simulink model "HydrogenRefuelingStation_Param"  (R2023b)
settings: Solver=VariableStepAuto  StartTime=0.0  StopTime=finSimulation  RelTol=1e-3  AbsTol=1e-3
PreLoadFcn:
  | load hydrogen_properties.mat
  | load silicone_fluid_properties.mat
  | 
  | p_storage = 200; % [bar]
  | p_vehicle_init = 100; % [bar]
  | T_env = 25; % [degC]
  | T_fluid = -60; % [degC]
  | 
  | V_vehicle = 172; % [l]
  | 
  | tube_D = 0.04; % [m]
  | hose_D = 0.0064; % [m]
  | pipe_D = 0.1; % [m]
  | 
  | num_buffer = 2;
  | 
  | intercooler_num_tubes = 25;
  | intercooler_tube_D = 0.008; % [m]
  | intercooler_shell_D = 0.1; % [m]
  | intercooler_L = 2; % [m]
  | 
  | precooler_tube_W = 0.001; % [m]
  | precooler_num_tubes = 50*25;
  | precooler_L = 1; % [m]
values from neighbouring files (symbols this model uses):
  EngDemandTime = 3000    [launch.m]
  EngThrottle = 1    [launch.m]
  ext_bufferEng_D = 0.025    [System_Parameters.m]
  ext_Manifold_D = 0.007    [System_Parameters.m]
  ext_vehTank_D = 0.25    [System_Parameters.m]
  in_bufferEng_D = 0.0064    [System_Parameters.m]
  in_Eng_D = 0.0064    [System_Parameters.m]
  in_Man_D = 0.0064    [System_Parameters.m]
  inOut_vehTank_D = 0.0064    [System_Parameters.m]
  int_bufferEng_D = 0.024    [System_Parameters.m]
  int_Manifold_D = 0.0064    [System_Parameters.m]
  int_vehTank_D = 0.22    [System_Parameters.m]
  L_bufferEng = 1    [System_Parameters.m]
  L_Manifold = 1    [System_Parameters.m]
  L_vehTank = 2    [System_Parameters.m]
  MV_D = 0.0064    [System_Parameters.m]
  out_bufferEng_D = 0.0064/2    (= 0.0032)    [System_Parameters.m]
  out_Eng_D = 0.0064    [System_Parameters.m]
  out_Man_D = 0.0064    [System_Parameters.m]
  Pipe_ConnMan_D = 0.0064    [System_Parameters.m]
  Pipe_ManPR_D = 0.0064    [System_Parameters.m]
  Pipe_ManTank_D = 0.0064    [System_Parameters.m]
  Pipe_PRBuffer_D = 0.0064    [System_Parameters.m]
  redn_PR_D = 0.0064    [System_Parameters.m]
  redn_PR_setP = 160    [System_Parameters.m]
  relief_PR_D = 0.0064    [System_Parameters.m]
  relief_vehTank_D = 0.0064    [System_Parameters.m]
  silicone_fluid =     [silicone_fluid_properties.mat]
  statConn_D = 0.0064    [System_Parameters.m]
  stationTrigger_Time = 2400    [System_Parameters.m]
  SV_D = 0.0064    [System_Parameters.m]
  tank_Man_D = 0.0064    [System_Parameters.m]
  TempCont_vehTank_D = 0.0064    [System_Parameters.m]
  vehConn_D = 0.0064    [System_Parameters.m]
  WP_high = 700    [System_Parameters.m]
libraries: fl_lib x128, nesl_utility x60, SimscapeFluids_lib x41, slpidlib x4
(part 1 of 6)
CloseFcn:
  | try,close(h1_HydrogenRefuelingStation),end
  | clear h1_HydrogenRefuelingStation
  | try,close(h2_HydrogenRefuelingStation),end
  | clear h2_HydrogenRefuelingStation
  | try,close(h3_HydrogenRefuelingStation),end
  | clear h3_HydrogenRefuelingStation
  | 
  | clear tout simlog_HydrogenRefuelingStation
  | clear H2 silicone_fluid
  | clear p_storage p_vehicle_init T_env T_fluid
  | clear V_vehicle tube_D hose_D pipe_D num_buffer
  | clear intercooler_num_tubes intercooler_tube_D intercooler_shell_D intercooler_L
  | clear precooler_tube_W precooler_num_tubes precooler_L
Description:
  | Hydrogen Refueling Station
settings Model: Creator=The MathWorks, Inc.  LastModifiedBy=sb74808
settings SolverCC: AutoScaleAbsTol=off  ZeroCrossAlgorithm=Adaptive  AlgebraicLoopSolver=TrustRegion  MaxZcPerStep=1
settings DataIOCC: ReturnWorkspaceOutputs=off
settings DebuggingCC: IgnoredZcDiagnostic=none  UnconnectedInputMsg=warning  UnconnectedOutputMsg=warning  UnconnectedLineMsg=warning  SymbolicDimsDataTypeCodeGenerationDiagnostic=none
settings ModelReferenceCC: EnableRefExpFcnMdlSchedulingChecks=on
settings SFSimCC: CustomCodeUndefinedFunction=UseInterfaceOnly
settings RTWCC: DLArmComputeVersion=19.05
settings SimscapeCC: SimscapeLogType=all  SimscapeLogSimulationStatistics=on  SimscapeLogName=simlog_HydrogenRefuelingStation  SimscapeLogDataHistory=10000

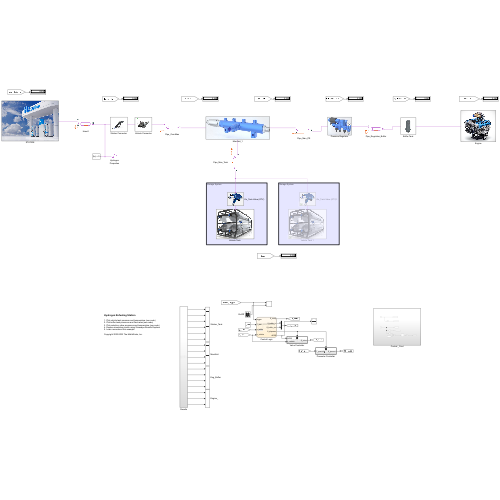
[thumbnail: Simulink's stored preview of the top-level diagram]
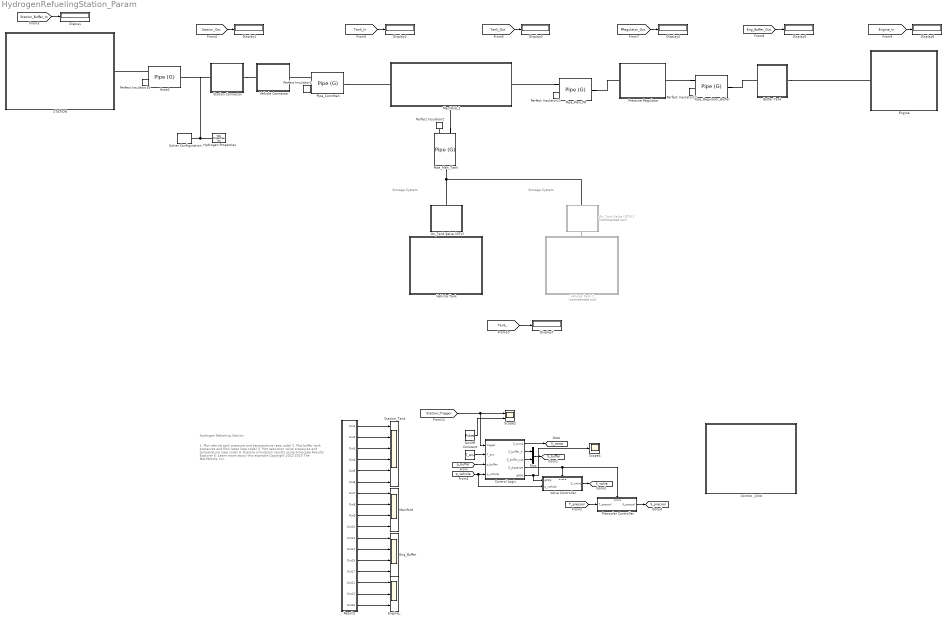
== system HydrogenRefuelingStation_Param ==
  note: Storage System
  note: Hydrogen Refueling Station
  note: 1. Plot vehicle tank pressure and temperature (see code)
      | 2. Plot buffer tank pressures and flow rates (see code)
      | 3. Plot reduction valve pressures and temperature (see code)
      | 4. Explore simulation results using Simscape Results Explorer
      | 5. Learn more about this example
      |
      | Copyright 2022-2023 The MathWorks, Inc.
  note: Storage System
  Buffer Tank : Subsystem
      mask Display: image('BufferTanks.png');
  Constant : Constant  Value=T_env
  Control Logic : Stateflow chart  Tag=PublishSubsystem  TreatAsAtomicUnit=on
      settings: PortSchema="{\"entries\":[{\"content\":{\"sides\":[{\"content\":{\"connectorIds\":[\"In4\",\"In1\",\"In2\",\"In3\"]},\"type\":\"ConnectorPlacement.EquallySpacedRectSide\",\"uuid\":\"229b392f-68ea-49e2-87d9-89899b0a8cf1\"},{\"content\":{\"connectorIds\":[\"Out2\",\"Out4\",\"Out5\",\"Out3\",\"Out1\"],\"side\":\"RIGHT\"},\"type\":\"ConnectorPlacement.EquallySpacedRectSide\",\"uuid\":\"67ffe3ee-1dc5-488d-9b3d-4fb771a503f6\"},{\"content\":{\"connectorIds\":[],\"side\":\"TOP\"},\"type\":\"ConnectorPlacement.EquallySpacedRectSide\",\"uuid\":\"803859aa-a920-419c-845f-f763b20f74de\"}]},\"type\":\"ConnectorPlacement.EquallySpacedConnector\",\"uuid\":\"a5c406d3-0f1f-4c42-8168-eaeee8551f27\"}],\"packageUris\":[\"http://schema.mathworks.com/mf0/Connector/R2020b\"],\"version\":\"1.0\"}"
  Control _Cmd : Subsystem
  Display{,1..7} (8 alike) : Display
  Eng_Buffer : Scope  NumInputPorts=4
  Engine : Subsystem
      mask Display: image('Engine_H2.PNG');
  Engine_ : Scope  NumInputPorts=3
  Hose2 : fl_lib/Gas/Elements/Pipe (G)  length=4 m  area=pi*statConn_D^2/4 m^2  Dh=statConn_D m  length_add=0.6 m  roughness=15e-6 m  Re_lam=2000  Re_tur=4000  shape_factor=64  Nu_lam=3.66  p_I_specify=on  p_I_priority=High  p_I=p_vehTank_init bar  p_I_nominal_specify=off  p_I_nominal_unit=MPa  p_I_nominal_value=1  T_I_specify=on  T_I_priority=High  T_I=T_env degC  T_I_nominal_specify=off  T_I_nominal_unit=K  T_I_nominal_value=1  rho_I_specify=off  rho_I_priority=None  rho_I=1.2 kg/m^3  rho_I_nominal_specify=off  rho_I_nominal_unit=kg/m^3  rho_I_nominal_value=1
  Hydrogen Properties : fl_lib/Gas/Utilities/Gas Properties (G)  gas_spec=foundation.enum.gas_spec.real_gas  R=0.287 kJ/(K*kg)  Z=1  T_ref=293.15 K  h_ref=420 kJ/kg  cp_ref=1 kJ/(K*kg)  mu_ref=18 s*uPa  k_ref=26 mW/(K*m)  T_TLU1=[150 : 10 : 200, 250 : 50 : 1000, 1500, 2000]' K  h_TLU1=[275.264783730547; 285.377054177734; 295.474578903607; 305.560871069627; 315.638490783961; 325.709373787179; 376.008033649461; 426.297784741196; 476.678788323875; 527.253890684429; 578.12722735187; 629.395040865183; 681.137690131207; 733.415442873049; 786.267894376777; 839.715851152006; 893.764459999509; 948.406676876931; 1003.62653219711; 1059.40193232821; 1115.70691941005; 1172.51341226958; 1762.18512007361; 2377.14064127409] kJ/kg  cp_TLU1=[1.01211492398124; 1.01042105529234; 1.00914159006373; 1.00815898273273; 1.00739688341918; 1.00680484569075; 1.00554191216852; 1.00637389921747; 1.0092105862442; 1.01414404435034; 1.02111299587909; 1.02986878923959; 1.04003820504128; 1.05120320041448; 1.06296312852444; 1.07497111709439; 1.08694865668905; 1.0986858495625; 1.11003396604319; 1.12089493621399; 1.13121051694521; 1.14095251451866; 1.21001953144; 1.24628356718428] kJ/(K*kg)  mu_TLU1=[10.3766056544352; 10.9908682444892; 11.5932000841352; 12.1841060353213; 12.764067709023; 13.3335437107148; 16.038149065057; 18.5373404836509; 20.8671495114253; 23.0554226800681; 25.1239717991959; 27.0901379793485; 28.96790749834; 30.7687111230031; 32.5020036481173; 34.17569027566; 35.7964450415303; 37.3699520751368; 38.9010908824946; 40.3940804368247; 41.8525925389218; 43.279841956487; 56.3254722619962; 68.068290080945] s*uPa  k_TLU1=[14.1517155766309; 15.0474512994325; 15.9300520513026; 16.7998749295306; 17.6573089963228; 18.5027588910197; 22.5644026699512; 26.384465676638; 30.0032801168886; 33.4532006033488; 36.7600619429332; 39.9446251241844; 43.0237448740114; 46.0112537033799; 48.9186234516389; 51.7554617696538; 54.5298878921773; 57.2488200454925; 59.9181976996146; 62.5431553064749; 65.128159527924; 67.6771186900213; 91.7815514375552; 114.486299090693] mW/(K*m)  T_TLU2=H2.T K  p_TLU2=H2.p MPa  rho_TLU2=H2.rho kg/m^3  s_TLU2=H2.s kJ/(K*kg)  h_TLU2=H2.h kJ/kg  cp_TLU2=H2.cp kJ/(K*kg)  mu_TLU2=H2.mu s*uPa  k_TLU2=H2.k mW/(K*m)  beta_TLU2=H2.beta MPa  alpha_TLU2=H2.alpha 1/K  T_min_perfect=1 K  T_max_perfect=inf K  p_min_perfect=1 Pa  p_max_perfect=inf MPa  T_range_flag=foundation.enum.T_range_G.from_props  T_min_semiperfect=150 K  T_max_semiperfect=2000 K  p_min_semiperfect=1 Pa  p_max_semiperfect=inf MPa  pT_region_flag=foundation.enum.pT_region_G.from_props  pT_validity_TLU2=ones(24, 20)  T_min_real=150 K  T_max_real=2000 K  p_min_real=0.001 MPa  p_max_real=10 MPa  p_atm=0.101325 MPa  properties_range_check=simscape.enum.assert.action.error  Mach_rev=0.001 / 10
  Manifold : Scope  NumInputPorts=4
  Manifold_1 : Subsystem  Tag=PublishSubsystem
      settings: PortSchema="{\"entries\":[{\"content\":{\"sides\":[{\"content\":{\"connectorIds\":[\"LConn1\"]},\"type\":\"ConnectorPlacement.EquallySpacedRectSide\",\"uuid\":\"b00ba4dd-6dda-4fc1-8418-16d977b72658\"},{\"content\":{\"connectorIds\":[\"RConn1\"],\"side\":\"RIGHT\"},\"type\":\"ConnectorPlacement.EquallySpacedRectSide\",\"uuid\":\"8ce3b878-20da-4ae3-b32b-b25a417e40c7\"},{\"content\":{\"side\":\"TOP\"},\"type\":\"ConnectorPlacement.EquallySpacedRectSide\",\"uuid\":\"178fea87-568c-460e-ad58-627cda0af208\"},{\"content\":{\"connectorIds\":[\"RConn2\"],\"side\":\"BOTTOM\"},\"type\":\"ConnectorPlacement.EquallySpacedRectSide\",\"uuid\":\"da377dea-32af-4e40-bf21-9605c244d1e1\"}]},\"type\":\"ConnectorPlacement.EquallySpacedConnector\",\"uuid\":\"9a70e3bb-46a6-4db7-b9e8-afd83bfe5c73\"}],\"packageUris\":[\"http://schema.mathworks.com/mf0/Connector/R2020b\"],\"version\":\"1.0\"}"
      mask Display: image('Manifold.jpg');
  Mux : Mux  Inputs=2
  On/Off : DiscretePulseGenerator  PulseType=Time based  Period=3600  PulseWidth=300 / 3600 * 100  PhaseDelay=2400
  On_Tank Valve (OTV) : Subsystem
      settings: PortSchema="{\"entries\":[{\"content\":{\"sides\":[{\"content\":{},\"type\":\"ConnectorPlacement.EquallySpacedRectSide\",\"uuid\":\"9d4661ff-bfd9-4877-b119-c7ad3b9158b6\"},{\"content\":{\"side\":\"RIGHT\"},\"type\":\"ConnectorPlacement.EquallySpacedRectSide\",\"uuid\":\"403ca504-bf4e-462a-96fb-b4ae1a4b51b2\"},{\"content\":{\"connectorIds\":[\"LConn1\"],\"side\":\"TOP\"},\"type\":\"ConnectorPlacement.EquallySpacedRectSide\",\"uuid\":\"f4930e4d-a2e3-4901-b32b-f7ec2035bb63\"},{\"content\":{\"connectorIds\":[\"RConn1\"],\"side\":\"BOTTOM\"},\"type\":\"ConnectorPlacement.EquallySpacedRectSide\",\"uuid\":\"d9d264b6-0917-42e9-93e5-2bb8167430bf\"}]},\"type\":\"ConnectorPlacement.EquallySpacedConnector\",\"uuid\":\"c2399e2b-f5dd-4ca5-8bb9-d4f6c8dace36\"}],\"packageUris\":[\"http://schema.mathworks.com/mf0/Connector/R2020b\"],\"version\":\"1.0\"}"
      mask Display: image('OTV.png');
  On_Tank Valve (OTV)1 : Subsystem  Commented=on
      settings: PortSchema="{\"entries\":[{\"content\":{\"sides\":[{\"content\":{},\"type\":\"ConnectorPlacement.EquallySpacedRectSide\",\"uuid\":\"9d4661ff-bfd9-4877-b119-c7ad3b9158b6\"},{\"content\":{\"side\":\"RIGHT\"},\"type\":\"ConnectorPlacement.EquallySpacedRectSide\",\"uuid\":\"403ca504-bf4e-462a-96fb-b4ae1a4b51b2\"},{\"content\":{\"connectorIds\":[\"LConn1\"],\"side\":\"TOP\"},\"type\":\"ConnectorPlacement.EquallySpacedRectSide\",\"uuid\":\"f4930e4d-a2e3-4901-b32b-f7ec2035bb63\"},{\"content\":{\"connectorIds\":[\"RConn1\"],\"side\":\"BOTTOM\"},\"type\":\"ConnectorPlacement.EquallySpacedRectSide\",\"uuid\":\"d9d264b6-0917-42e9-93e5-2bb8167430bf\"}]},\"type\":\"ConnectorPlacement.EquallySpacedConnector\",\"uuid\":\"c2399e2b-f5dd-4ca5-8bb9-d4f6c8dace36\"}],\"packageUris\":[\"http://schema.mathworks.com/mf0/Connector/R2020b\"],\"version\":\"1.0\"}"
      mask Display: image('OTV.png');
  Perfect Insulator{1..2,10..12} (5 alike) : fl_lib/Thermal/Thermal Elements/Perfect Insulator  T_specify=off  T_priority=None  T=293.15 K  T_nominal_specify=off  T_nominal_unit=K  T_nominal_value=1
  Pipe_ConnMan : fl_lib/Gas/Elements/Pipe (G)  length=Pipe_ConnMan_L m  area=pi*Pipe_ConnMan_D^2/4 m^2  Dh=Pipe_ConnMan_D m  length_add=0.6 m  roughness=15e-6 m  Re_lam=2000  Re_tur=4000  shape_factor=64  Nu_lam=3.66  p_I_specify=on  p_I_priority=High  p_I=p_vehTank_init bar  p_I_nominal_specify=off  p_I_nominal_unit=MPa  p_I_nominal_value=1  T_I_specify=on  T_I_priority=High  T_I=T_env degC  T_I_nominal_specify=off  T_I_nominal_unit=K  T_I_nominal_value=1  rho_I_specify=off  rho_I_priority=None  rho_I=1.2 kg/m^3  rho_I_nominal_specify=off  rho_I_nominal_unit=kg/m^3  rho_I_nominal_value=1
  Pipe_Man_PR : fl_lib/Gas/Elements/Pipe (G)  length=Pipe_ManPR_L m  area=pi*Pipe_ManPR_D^2/4 m^2  Dh=Pipe_ManPR_D m  length_add=0.6 m  roughness=15e-6 m  Re_lam=2000  Re_tur=4000  shape_factor=64  Nu_lam=3.66  p_I_specify=on  p_I_priority=High  p_I=p_vehTank_init bar  p_I_nominal_specify=off  p_I_nominal_unit=MPa  p_I_nominal_value=1  T_I_specify=on  T_I_priority=High  T_I=T_env degC  T_I_nominal_specify=off  T_I_nominal_unit=K  T_I_nominal_value=1  rho_I_specify=off  rho_I_priority=None  rho_I=1.2 kg/m^3  rho_I_nominal_specify=off  rho_I_nominal_unit=kg/m^3  rho_I_nominal_value=1
  Pipe_Man_Tank : fl_lib/Gas/Elements/Pipe (G)  length=Pipe_ManTank_L m  area=pi*Pipe_ManTank_D^2/4 m^2  Dh=Pipe_ManTank_D m  length_add=0.6 m  roughness=15e-6 m  Re_lam=2000  Re_tur=4000  shape_factor=64  Nu_lam=3.66  p_I_specify=on  p_I_priority=High  p_I=p_vehTank_init bar  p_I_nominal_specify=off  p_I_nominal_unit=MPa  p_I_nominal_value=1  T_I_specify=on  T_I_priority=High  T_I=T_env degC  T_I_nominal_specify=off  T_I_nominal_unit=K  T_I_nominal_value=1  rho_I_specify=off  rho_I_priority=None  rho_I=1.2 kg/m^3  rho_I_nominal_specify=off  rho_I_nominal_unit=kg/m^3  rho_I_nominal_value=1
  Pipe_Regulator_Buffer : fl_lib/Gas/Elements/Pipe (G)  length=Pipe_PRBuffer_L m  area=pi*Pipe_PRBuffer_D^2/4 m^2  Dh=Pipe_PRBuffer_D m  length_add=0.6 m  roughness=15e-6 m  Re_lam=2000  Re_tur=4000  shape_factor=64  Nu_lam=3.66  p_I_specify=on  p_I_priority=High  p_I=p_vehTank_init bar  p_I_nominal_specify=off  p_I_nominal_unit=MPa  p_I_nominal_value=1  T_I_specify=on  T_I_priority=High  T_I=T_env degC  T_I_nominal_specify=off  T_I_nominal_unit=K  T_I_nominal_value=1  rho_I_specify=off  rho_I_priority=None  rho_I=1.2 kg/m^3  rho_I_nominal_specify=off  rho_I_nominal_unit=kg/m^3  rho_I_nominal_value=1
  Precooler Controller : Subsystem  Tag=PublishSubsystem  TreatAsAtomicUnit=on
  Pressure Regulator : Subsystem
      mask Display: image('PressureRegulator.jpg');
  Results : Subsystem
  STATION : Subsystem
      mask Display: image('Hydrogen_Station_.png');
  Scope2 : Scope  NumInputPorts=2
  Scope4 : Scope
  Solver Configuration : nesl_utility/Solver Configuration  PhysicalDomain=network_engine_domain  SubClassName=solver  LeftPortType=input  RightPortType=generic  Tones=[]  Harmonics=[]  SimulateNoise=off  Profile=off  UseLocalSampling=off  EnableSwitchedLinearOptims=on  FrequencyDomain=off  UseCCode=off  RelTol=0.001  AbsTol=0.001  MinStep=1e-09  ToWorkspace=off  RevertToSquareIcSolve=off  NumHomotopyIterations=100  PhasorMode=off  PhasorModeNumHarmonics=1  ConsistencySolver=NEWTON_XTOL_AFTER_FTOL  IndexReductionMethod=DerivativeReplacement  DoDC=off  ResidualTolerance=1e-09  ConsistencyTolSource=GLOBAL  ConsistencyAbsTol=0.001  ConsistencyRelTol=0.001  ConsistencyTolFactor=0.001  UseLocalSolver=off  LocalSolverChoice=NE_BACKWARD_EULER_ADVANCER  ResolveIndetEquations=on  FunctionEvalNumThread=1  LocalSolverSampleTime=0.001  DoFixedCost=off  MaxNonlinIter=3  MaxModeIter=2  ComputeImpulses=off  ImpulseIterations=2  LinearAlgebra=auto  LinearAlgebraNumThread=0  EquationFormulation=NE_TIME_EF  DelaysMemoryBudget=1024  AutomaticFiltering=on  FilteringTimeConstant=0.001  PartitionStorageMethod=AS_NEEDED  PartitionMemoryBudget=1024  PartitionMethod=ROBUST  MultibodyUseLocalSolver=off  MultibodyLocalSolverChoice=ODE1  MultibodyLocalSolverSampleTime=0.001
  Station Connector : Subsystem
      mask Display: image('FuelingNozzle.png');
  Station_Tank : Scope  NumInputPorts=6
  Valve Controller : Subsystem  Tag=PublishSubsystem  TreatAsAtomicUnit=on
  Vehicle Connector : Subsystem
      mask Display: image('Veh_Connector.jpg');
  "Vehicle Tank " : Subsystem
      mask Display: image('Vehicle_Tank.png');
  Vehicle Tank 1 : Subsystem  Commented=on
      mask Display: image('Vehicle_Tank.png');
  tag scope: S_buffer=global, S_comp=global, S_precool=global, S_valve=global
  wires:
  Constant/1 -> Control Logic/1(T_env)
  [Station_Trigger] -> Control Logic/4(trigger), Scope2/1
  Control Logic/3(S_dispense) -> Valve Controller/Enable, Precooler Controller/Enable
  Control Logic/1(APRR) -> Scope4/1, Valve Controller/1(APRR)
  [p_buffer] -> Control Logic/2(p_buffer)
  [p_vehicle] -> Valve Controller/2(p_vehicle), Control Logic/3(p_vehicle)
  Control Logic/2(S_comp) -> [S_comp]
  Control Logic/4(S_buffer_in) -> Mux/1
  Control Logic/5(S_buffer_out) -> Mux/2
  Valve Controller/1(S_valve) -> [S_valve]
  Precooler Controller/1(S_precool) -> [S_precool]
  [T_precool] -> Precooler Controller/1(T_precool)
  Mux/1 -> [S_buffer]
  Results/1(Out1) -> Station_Tank/1
  Results/2(Out2) -> Station_Tank/2
  Results/3(Out3) -> Station_Tank/3
  Results/4(Out4) -> Station_Tank/4
  Results/5(Out5) -> Station_Tank/5
  Results/6(Out6) -> Station_Tank/6
  Results/7(Out7) -> Manifold/1
  Results/8(Out8) -> Manifold/2
  Results/9(Out9) -> Manifold/3
  Results/10(Out10) -> Manifold/4
  Results/15(Out11) -> Engine_/1
  Results/16(Out12) -> Engine_/2
  Results/11(Out13) -> Eng_Buffer/1
  Results/12(Out14) -> Eng_Buffer/2
  Results/13(Out15) -> Eng_Buffer/3
  Results/17(Out16) -> Engine_/3
  [Station_Buffer_In] -> Display/1
  [Station_Out] -> Display1/1
  [Tank_In] -> Display2/1
  [Tank_Out] -> Display3/1
  [PRegulator_Out] -> Display4/1
  [Eng_Buffer_Out] -> Display5/1
  [Engine_In] -> Display6/1
  [Tank_] -> Display7/1
  Results/14(Out17) -> Eng_Buffer/4
  On/Off/1 -> Scope2/2
  connections:
  Hydrogen Properties/RConn1 -- Station Connector/LConn1 -- Hose2/RConn1 -- Solver Configuration/RConn1
  Pipe_Man_Tank/RConn1 -- On_Tank Valve (OTV)1/LConn1 -- On_Tank Valve (OTV)/LConn1
  Perfect Insulator10/LConn1 -- Hose2/LConn2
  Perfect Insulator11/LConn1 -- Pipe_Man_PR/LConn2
  Pipe_Man_PR/LConn1 -- Manifold_1/RConn1
  Pipe_Man_PR/RConn1 -- Pressure Regulator/LConn1
  Pipe_Regulator_Buffer/LConn1 -- Pressure Regulator/RConn1
  Perfect Insulator12/LConn1 -- Pipe_Regulator_Buffer/LConn2
  Pipe_ConnMan/RConn1 -- Manifold_1/LConn1
  Perfect Insulator1/LConn1 -- Pipe_ConnMan/LConn2
  Pipe_ConnMan/LConn1 -- Vehicle Connector/RConn1
  Hose2/LConn1 -- STATION/RConn1
  Station Connector/RConn1 -- Vehicle Connector/LConn1
  On_Tank Valve (OTV)/RConn1 -- "Vehicle Tank "/LConn1
  Pipe_Regulator_Buffer/RConn1 -- Buffer Tank/LConn1
  Buffer Tank/RConn1 -- Engine/LConn1
  Perfect Insulator2/LConn1 -- Pipe_Man_Tank/LConn2
  Pipe_Man_Tank/LConn1 -- Manifold_1/RConn2
  On_Tank Valve (OTV)1/RConn1 -- Vehicle Tank 1/LConn1

== system HydrogenRefuelingStation_Param/Buffer Tank ==
  Buffer Tank : Subsystem
      settings: PortSchema="{\"entries\":[{\"content\":{\"sides\":[{\"content\":{\"connectorIds\":[\"LConn1\"]},\"type\":\"ConnectorPlacement.EquallySpacedRectSide\",\"uuid\":\"be55c30a-ebc5-4db6-8bf5-c32b00e208a6\"},{\"content\":{\"connectorIds\":[\"RConn1\"],\"side\":\"RIGHT\"},\"type\":\"ConnectorPlacement.EquallySpacedRectSide\",\"uuid\":\"32ce90ed-16b2-412b-9043-f12374b22354\"},{\"content\":{\"connectorIds\":[\"Out1\",\"Out2\",\"Out3\",\"Out4\"],\"side\":\"TOP\"},\"type\":\"ConnectorPlacement.EquallySpacedRectSide\",\"uuid\":\"f980e63f-25af-4287-a163-12bb2aff40ef\"}]},\"type\":\"ConnectorPlacement.EquallySpacedConnector\",\"uuid\":\"15029ed0-97ce-4ec5-8ed4-a10d8c49a03a\"}],\"packageUris\":[\"http://schema.mathworks.com/mf0/Connector/R2020b\"],\"version\":\"1.0\"}"
  A : PMIOPort  Side=Left
  B : PMIOPort  Port=2  Side=Right
  tag scope: T_Buffer_Eng=global, m_Buffer_Eng_In=global, m_Buffer_Eng_Out=global, p_Buffer_Eng=global
  wires:
  Buffer Tank/1(p_Buffer_Eng) -> [p_Buffer_Eng]
  Buffer Tank/2(m_Buffer_Eng_In) -> [m_Buffer_Eng_In]
  Buffer Tank/3(m_Buffer_Eng_Out) -> [m_Buffer_Eng_Out]
  Buffer Tank/4(T_Buffer_Eng) -> [T_Buffer_Eng]
  connections:
  Buffer Tank/RConn1 -- B/RConn1
  A/RConn1 -- Buffer Tank/LConn1

== system HydrogenRefuelingStation_Param/Control Logic/SAE_J2601 ==
  T_env : Inport  OutDataTypeStr=double  PortDimensions=1
  p_init : Inport  Port=2  OutDataTypeStr=double  PortDimensions=1
  f : TriggerPort  TriggerType=function-call  VariantControl=(inherit)
      settings: CopyFcn=Stateflow.SLINSF.SimulinkMan.removeBlockPreDeleteFcn  PreDeleteFcn=Stateflow.SLINSF.SimulinkMan.unsafePredeleteFcn
  APRR [MPa/min] : Lookup_n-D  NumberOfTableDimensions=1  BreakpointsForDimension1=[-41;-40;-30;-20;-10;0;10;20;25;30;35;40;45;50;51]  Table=[0;28.5;28.5;28.5;28.5;28.5;28;21.8;18.5;15.3;12.4;11.5;8.1;5.1;0]  InterpMethod=Nearest  InternalRulePriority=Speed  RndMeth=Simplest
  MPa to bar : Gain  Gain=10
  MPa/min to bar/s : Gain  Gain=1/6
  Scope : Scope  NumInputPorts=4
  Target Pressure [MPa] : Lookup_n-D  BreakpointsForDimension1=[-41;-40;-30;-20;-10;0;10;20;25;30;35;40;45;50;51]  BreakpointsForDimension2=[0.4;0.5;2;5;10;15;20;30;40;50;60;70;71]  Table=[0 0 0 0 0 0 0 0 0 0 0 0 0;0 71.6 71.1 70.2 70 68.5 66.9 64.8 61.5 58.5 0 0 0;0 72.1 71.6 70.6 70.4 69 67.4 65.2 61.8 58.7 0 0 0;0 72.9 72.3 71.3 71 69.5 68 65.7 62.4 60 0 0 0;0 73.4 72.9 71.9 70 70 68.4 66.5 64.4 62.9 61.2 0 0;0 74 73.4 72.4 70.6 70.7 69.6 68.6 67.1 65.7 64 0 0;0 66.3 71.1 74.1 73.2 72.4 71.6 70.9 69.6 68.4 66.9 0 0;0 67.9 72.1 74.5 73.7 74 73.4 72.2 71.9 70.7 69.7 0 0;0 69 72.8 75.1 74.5 74.7 74.3 73.3 73 72 71.1 0 0;0 70.6 73.9 75.8 75.2 75.4 75.1 74.3 74.1 73.3 72.4 71.3 0;0 72.9 75.3 76.4 76 76.1 75.9 75.3 75.1 74.5 73.8 72.7 0;0 73.2 75.6 76.8 76.3 76.4 76.2 75.6 75.3 74.6 73.9 72.7 0;0 76.3 77.2 76.9 76.5 76.4 76.2 75.6 75.3 74.7 73.9 72.7 0;0 77.8 77.6 77.3 76.9 76.6 76.2 75.7 75.3 74.7 73.9 72.8 0;0 0 0 0 0 0 0 0 0 0 0 0 0]  InterpMethod=Nearest  InternalRulePriority=Speed  RndMeth=Simplest
      settings: InputPortMap=u0,u1
  bar to MPa : Gain  Gain=0.1
  APRR : Outport
  p_target : Outport  Port=2
  wires:
  bar to MPa/1 -> Scope/3, Target Pressure [MPa]/2
  T_env/1 -> Scope/1, Target Pressure [MPa]/1, APRR [MPa/min]/1
  p_init/1 -> bar to MPa/1
  APRR [MPa/min]/1 -> Scope/2, MPa/min to bar/s/1
  Target Pressure [MPa]/1 -> Scope/4, MPa to bar/1
  MPa/min to bar/s/1 -> APRR/1
  MPa to bar/1 -> p_target/1

== system HydrogenRefuelingStation_Param/Control _Cmd ==
  Constant : Constant  Value=EngThrottle
  Delay : Delay  DelayLength=1
  Delay1 : Delay
  Delay2 : Delay  DelayLength=1
  Eng_Tank_Out1 : Step  Time=EngDemandTime  SampleTime=0.5
  Engine Massflow control : Lookup_n-D  NumberOfTableDimensions=1  BreakpointsForDimension1=[0 1 2 3 4 5]  Table=[0 3.29 4.39 5.31 6.26 6.92]  ExtrapMethod=Clip  InternalRulePriority=Speed  RndMeth=Simplest
  Gain3 : Gain  Gain=1e-3
  On/Off1 : DiscretePulseGenerator  PulseType=Time based  Period=3600  PulseWidth=300 / 3600 * 100  PhaseDelay=stationTrigger_Time
  Product : Product
  tag scope: Eng_Buffer_Valve_Cmd=global, Eng_Ctrl=global, Station_Trigger=global, Tank_In_cmd=global, Tank_Out_cmd=global
  wires:
  Product/1 -> Engine Massflow control/1
  Gain3/1 -> [Eng_Ctrl]
  Engine Massflow control/1 -> Gain3/1
  On/Off1/1 -> [Station_Trigger], Delay/1
  Delay/1 -> [Tank_In_cmd]
  Eng_Tank_Out1/1 -> Delay1/1, Delay2/1, [Tank_Out_cmd]
  Delay2/1 -> [Eng_Buffer_Valve_Cmd]
  Delay1/1 -> Product/1
  Constant/1 -> Product/2

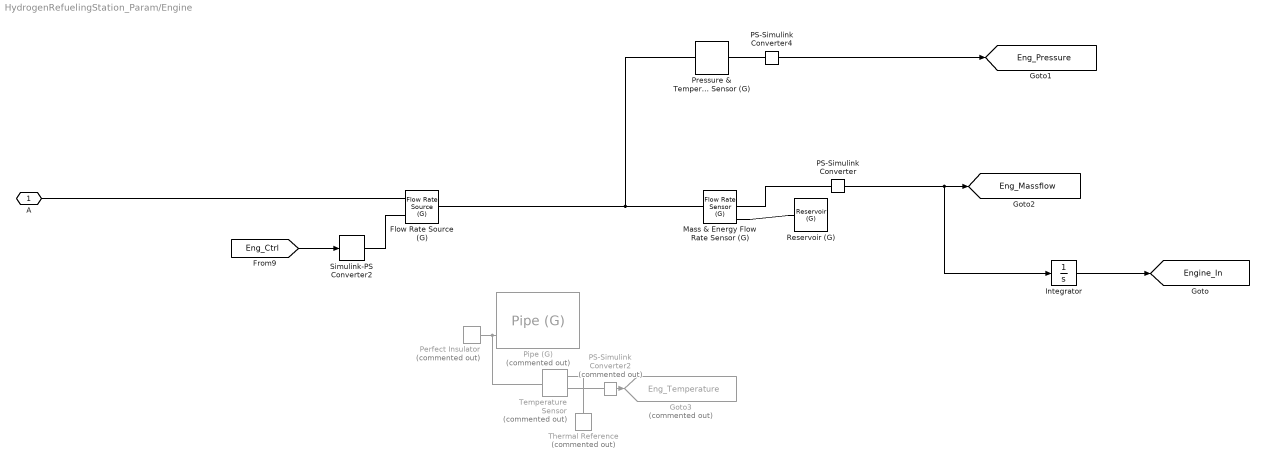
== system HydrogenRefuelingStation_Param/Engine ==
  Flow Rate Source (G) : fl_lib/Gas/Sources/Flow Rate Source (G)  source_type=foundation.enum.constant_controlled.controlled  flow_type=foundation.enum.mass_volumetric_flow.mass  mass_flow=0 kg/s  volumetric_flow=0 m^3/s  volumetric_flow_conditions=foundation.enum.volumetric_flow_conditions.actual  p_std=0.101325 MPa  T_std=20 degC  power_spec=foundation.enum.power_spec.none  area_A=pi*in_Eng_D^2/4 m^2  area_B=pi*out_Eng_D^2/4 m^2
      settings: InternalSimscapePortConfiguration="{\"Bottom\":[],\"Left\":[{\"id\":\"A\",\"label\":\"A\",\"type\":\"foundation.gas.gas\"},{\"id\":\"M\",\"label\":\"M\",\"type\":\"input\"}],\"Right\":[{\"id\":\"B\",\"label\":\"B\",\"type\":\"foundation.gas.gas\"}],\"Top\":[]}"
  Goto3 : Goto  Commented=on  GotoTag=Eng_Temperature  TagVisibility=global
  Integrator : Integrator
  Mass & Energy Flow Rate Sensor (G) : fl_lib/Gas/Sensors/Flow Rate Sensor (G)  mass_flow_measure=true  volumetric_flow_measure=false  volumetric_flow_conditions=foundation.enum.volumetric_flow_conditions.actual  p_std=0.101325 MPa  T_std=20 degC  energy_flow_measure=true
      settings: InternalSimscapePortConfiguration="{\"Bottom\":[{\"id\":\"PHI\",\"label\":\"φ\",\"type\":\"output\"}],\"Left\":[{\"id\":\"A\",\"label\":\"A\",\"type\":\"foundation.gas.gas\"}],\"Right\":[{\"id\":\"B\",\"label\":\"B\",\"type\":\"foundation.gas.gas\"},{\"id\":\"M\",\"label\":\"M\",\"type\":\"output\"}],\"Top\":[]}"
  PS-Simulink Converter : nesl_utility/PS-Simulink Converter  PhysicalDomain=network_engine_domain  SubClassName=ps_output  LeftPortType=input  RightPortType=output  PseudoPeriodic=off  Frequencies=[]  VectorFormat=inherit  Unit=kg/s  AffineConversion=off
  PS-Simulink Converter2 : nesl_utility/PS-Simulink Converter  Commented=on  PhysicalDomain=network_engine_domain  SubClassName=ps_output  LeftPortType=input  RightPortType=output  PseudoPeriodic=off  Frequencies=[]  VectorFormat=inherit  Unit=degC  AffineConversion=on
  PS-Simulink Converter4 : nesl_utility/PS-Simulink Converter  PhysicalDomain=network_engine_domain  SubClassName=ps_output  LeftPortType=input  RightPortType=output  PseudoPeriodic=off  Frequencies=[]  VectorFormat=inherit  Unit=bar  AffineConversion=off
  Perfect Insulator : fl_lib/Thermal/Thermal Elements/Perfect Insulator  Commented=on  T_specify=off  T_priority=None  T=293.15 K  T_nominal_specify=off  T_nominal_unit=K  T_nominal_value=1
  Pipe (G) : fl_lib/Gas/Elements/Pipe (G)  Commented=on  length=0.1 m  area=(pi*hose_D^2/6) m^2  Dh=hose_D m  length_add=0.1 m  roughness=15e-6 m  Re_lam=2000  Re_tur=4000  shape_factor=64  Nu_lam=3.66  p_I_specify=off  p_I_priority=High  p_I=0.101325 MPa  p_I_nominal_specify=off  p_I_nominal_unit=MPa  p_I_nominal_value=1  T_I_specify=off  T_I_priority=High  T_I=293.15 K  T_I_nominal_specify=off  T_I_nominal_unit=K  T_I_nominal_value=1  rho_I_specify=off  rho_I_priority=None  rho_I=1.2 kg/m^3  rho_I_nominal_specify=off  rho_I_nominal_unit=kg/m^3  rho_I_nominal_value=1
  Pressure & Temperature Sensor (G) : fl_lib/Gas/Sensors/Pressure & Temperature Sensor (G)  reference=foundation.enum.MeasurementReference.absolute  pressure=true  pressure_spec=foundation.enum.PressureMeasementSpec.Absolute  temperature=false
      settings: InternalSimscapePortConfiguration="{\"Bottom\":[],\"Left\":[{\"id\":\"A\",\"label\":\"A\",\"type\":\"foundation.gas.gas\"}],\"Right\":[{\"id\":\"Pa\",\"label\":\"Pa\",\"type\":\"output\"}],\"Top\":[]}"
  Reservoir (G) : fl_lib/Gas/Elements/Reservoir (G)  pressure_spec=foundation.enum.pressure_spec.specified  reservoir_pressure=p_Eng bar  reservoir_temperature=T_Eng K  area_A=pi*out_Eng_D^2/4 m^2
  Simulink-PS Converter2 : nesl_utility/Simulink-PS Converter  PhysicalDomain=network_engine_domain  SubClassName=ps_input  LeftPortType=input  RightPortType=output  PseudoPeriodic=off  Frequencies=[]  NoiseDistribution=none  NoiseParameters=[]  Unit=kg/s  AffineConversion=off  FilteringAndDerivatives=provide  SimscapeFilterOrder=1  InputFilterTimeConstant=0.001  UdotUserProvided=0
  Temperature Sensor : fl_lib/Thermal/Thermal Sensors/Temperature Sensor  Commented=on  temperature_measure=foundation.enum.MeasurementReference.difference
  Thermal Reference : fl_lib/Thermal/Thermal Elements/Thermal Reference  Commented=on
  "A  " : PMIOPort  Side=Left
  tag scope: Eng_Massflow=global, Eng_Pressure=global, Engine_In=global
  wires:
  PS-Simulink Converter4/1 -> [Eng_Pressure]
  PS-Simulink Converter/1 -> Integrator/1, [Eng_Massflow]
  [Eng_Ctrl] -> Simulink-PS Converter2/1
  PS-Simulink Converter2/1 -> Goto3/1
  Integrator/1 -> [Engine_In]
  connections:
  Pressure & Temperature Sensor (G)/LConn1 -- Flow Rate Source (G)/RConn1 -- Mass & Energy Flow Rate Sensor (G)/LConn1
  Flow Rate Source (G)/LConn1 -- "A  "/RConn1
  Mass & Energy Flow Rate Sensor (G)/RConn1 -- Reservoir (G)/LConn1
  Simulink-PS Converter2/RConn1 -- Flow Rate Source (G)/LConn2
  PS-Simulink Converter/LConn1 -- Mass & Energy Flow Rate Sensor (G)/RConn2
  PS-Simulink Converter4/LConn1 -- Pressure & Temperature Sensor (G)/RConn1
  Pipe (G)/LConn2 -- Temperature Sensor/LConn1 -- Perfect Insulator/LConn1
  Temperature Sensor/RConn1 -- Thermal Reference/LConn1
  PS-Simulink Converter2/LConn1 -- Temperature Sensor/RConn2

== system HydrogenRefuelingStation_Param/Manifold_1 ==
  Subsystem : Subsystem
      settings: PortSchema="{\"entries\":[{\"content\":{\"sides\":[{\"content\":{\"connectorIds\":[\"LConn1\",\"In1\"]},\"type\":\"ConnectorPlacement.EquallySpacedRectSide\",\"uuid\":\"4c0af899-441c-4bee-a394-f4ebb3cc096d\"},{\"content\":{\"connectorIds\":[\"RConn1\"],\"side\":\"RIGHT\"},\"type\":\"ConnectorPlacement.EquallySpacedRectSide\",\"uuid\":\"331d1815-40f8-45df-887e-8493421d705f\"},{\"content\":{\"connectorIds\":[\"Out1\",\"Out2\",\"Out3\",\"Out4\",\"Out5\"],\"side\":\"TOP\"},\"type\":\"ConnectorPlacement.EquallySpacedRectSide\",\"uuid\":\"c706b27c-1d0a-403d-b00b-17d6f7f02715\"},{\"content\":{\"connectorIds\":[\"RConn2\"],\"side\":\"BOTTOM\"},\"type\":\"ConnectorPlacement.EquallySpacedRectSide\",\"uuid\":\"143dcec0-fee2-4dc6-a215-548477a4ebfa\"}]},\"type\":\"ConnectorPlacement.EquallySpacedConnector\",\"uuid\":\"71979b40-d65d-4478-96c5-a233c5950d54\"}],\"packageUris\":[\"http://schema.mathworks.com/mf0/Connector/R2020b\"],\"version\":\"1.0\"}"
  Manifold_In : PMIOPort  Side=Left
  Manifold_Out : PMIOPort  Port=2  Side=Right
  Tank : PMIOPort  Port=3  Side=Right
  tag scope: T_Manifold=global, m_Manifold_In=global, m_Manifold_Out=global, m_Manifold_Tank=global, p_Manifold=global
  wires:
  Subsystem/1(p_Manifold) -> [p_Manifold]
  Subsystem/5(T_Manifold) -> [T_Manifold]
  Subsystem/2(m_Man_In) -> [m_Manifold_In]
  Subsystem/3(m_Man_Tank_Eng) -> [m_Manifold_Tank]
  Subsystem/4(m_Tank_Out) -> [m_Manifold_Out]
  [Tank_Out_cmd] -> Subsystem/1(Tank_Out_cmd)
  connections:
  Subsystem/RConn2 -- Tank/RConn1
  Subsystem/LConn1 -- Manifold_In/RConn1
  Subsystem/RConn1 -- Manifold_Out/RConn1

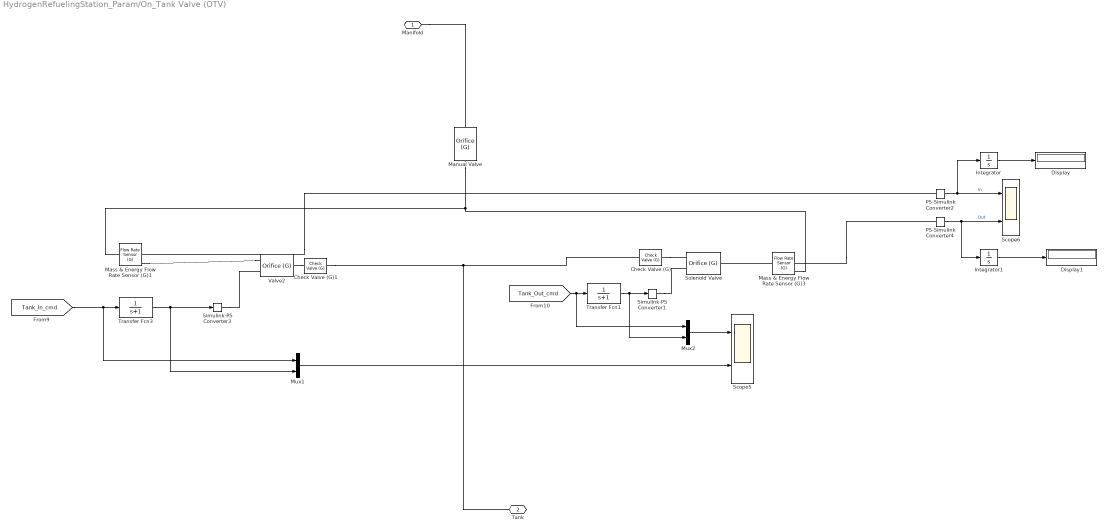
== system HydrogenRefuelingStation_Param/On_Tank Valve (OTV) ==
  Check Valve (G) : SimscapeFluids_lib/Gas/Valves & Orifices/Directional Control Valves/Check Valve (G)  opening_pressure_spec=fluids.gas.valves_orifices.enum.PressureControlSpec.PressureA  p_crack_differential=0.01 MPa  p_crack_gauge=1 bar  press_max_differential=70 MPa  press_max_gauge=WP_high bar  valve_parameterization=fluids.gas.valves_orifices.enum.OrificeParameterization.Cv  Cv_max=0.8  xT_Cv=0.7  Kv_max=3.6  xT_Kv=0.7  C_max=12 l/(bar*s)  B_crit_linear=0.3  m=0.5  T_ref_C=293.15 K  rho_ref_C=1.185 kg/m^3  orifice_area_max=1e-4 m^2  Cd=0.64  leakage_fraction=1e-6  smoothing_factor=0.01  B_lam=0.999  area=pi*MV_D ^2/4 m^2
      settings: InternalSimscapePortConfiguration="{\"Bottom\":[],\"Left\":[{\"id\":\"A\",\"label\":\"A\",\"type\":\"foundation.gas.gas\"}],\"Right\":[{\"id\":\"B\",\"label\":\"B\",\"type\":\"foundation.gas.gas\"}],\"Top\":[]}"
  Check Valve (G)1 : SimscapeFluids_lib/Gas/Valves & Orifices/Directional Control Valves/Check Valve (G)  opening_pressure_spec=fluids.gas.valves_orifices.enum.PressureControlSpec.PressureA  p_crack_differential=0.01 MPa  p_crack_gauge=1 bar  press_max_differential=70 MPa  press_max_gauge=WP_high bar  valve_parameterization=fluids.gas.valves_orifices.enum.OrificeParameterization.Cv  Cv_max=0.8  xT_Cv=0.7  Kv_max=3.6  xT_Kv=0.7  C_max=12 l/(bar*s)  B_crit_linear=0.3  m=0.5  T_ref_C=293.15 K  rho_ref_C=1.185 kg/m^3  orifice_area_max=1e-4 m^2  Cd=0.64  leakage_fraction=1e-6  smoothing_factor=0.01  B_lam=0.999  area=pi*MV_D ^2/4 m^2
      settings: InternalSimscapePortConfiguration="{\"Bottom\":[],\"Left\":[{\"id\":\"A\",\"label\":\"A\",\"type\":\"foundation.gas.gas\"}],\"Right\":[{\"id\":\"B\",\"label\":\"B\",\"type\":\"foundation.gas.gas\"}],\"Top\":[]}"
  Display : Display
  Display1 : Display
  Integrator : Integrator
  Integrator1 : Integrator
  Manual Valve : SimscapeFluids_lib/Gas/Valves & Orifices/Orifice (G)  orifice_type=foundation.enum.constant_variable.constant  orifice_parameterization=fluids.gas.valves_orifices.enum.OrificeParameterization.Cv  opening_characteristic=fluids.gas.valves_orifices.enum.OpeningCharacteristics.Linear  Cv_constant=4  Cv_max=4  L_Cv_TLU=0 : 0.2 : 1  Cv_TLU=[1e-06, .8, 1.6, 2.4, 3.2, 4]  xT_Cv=0.7  Kv_constant=3.6  Kv_max=3.6  L_Kv_TLU=0 : 0.2 : 1  Kv_TLU=[1e-06, .72, 1.44, 2.16, 2.88, 3.6]  xT_Kv=0.7  C_constant=12 l/(bar*s)  B_crit_constant=0.3  C_max=12 l/(bar*s)  B_crit_linear=0.3  L_C_TLU=0 : 0.2 : 1  C_TLU=[1e-05, 2.4, 4.8, 7.2, 9.6, 12] l/(bar*s)  B_crit_TLU=0.3 * ones(1, 6)  m=0.5  T_ref_C=293.15 K  rho_ref_C=1.185 kg/m^3  orifice_area_constant=1e-4 m^2  orifice_area_max=1e-4 m^2  L_orifice_area_TLU=0 : 0.2 : 1  orifice_area_TLU=[1e-10, 2e-05, 4e-05, 6e-05, 8e-05, .0001] m^2  Cd=0.64  leakage_fraction=1e-6  smoothing_factor=0  B_lam=0.999  area=pi*inOut_vehTank_D^2/4 m^2
      settings: InternalSimscapePortConfiguration="{\"Bottom\":[],\"Left\":[{\"id\":\"A\",\"label\":\"A\",\"type\":\"foundation.gas.gas\"}],\"Right\":[{\"id\":\"B\",\"label\":\"B\",\"type\":\"foundation.gas.gas\"}],\"Top\":[]}"
  Mass & Energy Flow Rate Sensor (G)1 : fl_lib/Gas/Sensors/Flow Rate Sensor (G)  mass_flow_measure=true  volumetric_flow_measure=false  volumetric_flow_conditions=foundation.enum.volumetric_flow_conditions.actual  p_std=0.101325 MPa  T_std=20 degC  energy_flow_measure=true
      settings: InternalSimscapePortConfiguration="{\"Bottom\":[{\"id\":\"PHI\",\"label\":\"φ\",\"type\":\"output\"}],\"Left\":[{\"id\":\"A\",\"label\":\"A\",\"type\":\"foundation.gas.gas\"}],\"Right\":[{\"id\":\"B\",\"label\":\"B\",\"type\":\"foundation.gas.gas\"},{\"id\":\"M\",\"label\":\"M\",\"type\":\"output\"}],\"Top\":[]}"
  Mass & Energy Flow Rate Sensor (G)3 : fl_lib/Gas/Sensors/Flow Rate Sensor (G)  mass_flow_measure=true  volumetric_flow_measure=false  volumetric_flow_conditions=foundation.enum.volumetric_flow_conditions.actual  p_std=0.101325 MPa  T_std=20 degC  energy_flow_measure=true
      settings: InternalSimscapePortConfiguration="{\"Bottom\":[{\"id\":\"PHI\",\"label\":\"φ\",\"type\":\"output\"}],\"Left\":[{\"id\":\"A\",\"label\":\"A\",\"type\":\"foundation.gas.gas\"}],\"Right\":[{\"id\":\"B\",\"label\":\"B\",\"type\":\"foundation.gas.gas\"},{\"id\":\"M\",\"label\":\"M\",\"type\":\"output\"}],\"Top\":[]}"
  Mux1 : Mux  Inputs=2
  Mux2 : Mux  Inputs=2
  PS-Simulink Converter2 : nesl_utility/PS-Simulink Converter  PhysicalDomain=network_engine_domain  SubClassName=ps_output  LeftPortType=input  RightPortType=output  PseudoPeriodic=off  Frequencies=[]  VectorFormat=inherit  Unit=kg/s  AffineConversion=off
  PS-Simulink Converter4 : nesl_utility/PS-Simulink Converter  PhysicalDomain=network_engine_domain  SubClassName=ps_output  LeftPortType=input  RightPortType=output  PseudoPeriodic=off  Frequencies=[]  VectorFormat=inherit  Unit=kg/s  AffineConversion=off
  Scope5 : Scope  NumInputPorts=2
  Scope6 : Scope  NumInputPorts=2
  Simulink-PS Converter1 : nesl_utility/Simulink-PS Converter  PhysicalDomain=network_engine_domain  SubClassName=ps_input  LeftPortType=input  RightPortType=output  PseudoPeriodic=off  Frequencies=[]  NoiseDistribution=none  NoiseParameters=[]  Unit=1  AffineConversion=off  FilteringAndDerivatives=provide  SimscapeFilterOrder=1  InputFilterTimeConstant=0.001  UdotUserProvided=0
  Simulink-PS Converter3 : nesl_utility/Simulink-PS Converter  PhysicalDomain=network_engine_domain  SubClassName=ps_input  LeftPortType=input  RightPortType=output  PseudoPeriodic=off  Frequencies=[]  NoiseDistribution=none  NoiseParameters=[]  Unit=1  AffineConversion=off  FilteringAndDerivatives=provide  SimscapeFilterOrder=1  InputFilterTimeConstant=0.001  UdotUserProvided=0
  Solenoid Valve : SimscapeFluids_lib/Gas/Valves & Orifices/Orifice (G)  orifice_type=foundation.enum.constant_variable.variable  orifice_parameterization=fluids.gas.valves_orifices.enum.OrificeParameterization.Cv  opening_characteristic=fluids.gas.valves_orifices.enum.OpeningCharacteristics.Linear  Cv_constant=4  Cv_max=4  L_Cv_TLU=0 : 0.2 : 1  Cv_TLU=[1e-06, .8, 1.6, 2.4, 3.2, 4]  xT_Cv=0.7  Kv_constant=3.6  Kv_max=3.6  L_Kv_TLU=0 : 0.2 : 1  Kv_TLU=[1e-06, .72, 1.44, 2.16, 2.88, 3.6]  xT_Kv=0.7  C_constant=12 l/(bar*s)  B_crit_constant=0.3  C_max=12 l/(bar*s)  B_crit_linear=0.3  L_C_TLU=0 : 0.2 : 1  C_TLU=[1e-05, 2.4, 4.8, 7.2, 9.6, 12] l/(bar*s)  B_crit_TLU=0.3 * ones(1, 6)  m=0.5  T_ref_C=293.15 K  rho_ref_C=1.185 kg/m^3  orifice_area_constant=1e-4 m^2  orifice_area_max=1e-4 m^2  L_orifice_area_TLU=0 : 0.2 : 1  orifice_area_TLU=[1e-10, 2e-05, 4e-05, 6e-05, 8e-05, .0001] m^2  Cd=0.64  leakage_fraction=1e-6  smoothing_factor=0  B_lam=0.999  area=pi*SV_D ^2/4 m^2
      settings: InternalSimscapePortConfiguration="{\"Bottom\":[],\"Left\":[{\"id\":\"A\",\"label\":\"A\",\"type\":\"foundation.gas.gas\"},{\"id\":\"L\",\"label\":\"L\",\"type\":\"input\"}],\"Right\":[{\"id\":\"B\",\"label\":\"B\",\"type\":\"foundation.gas.gas\"}],\"Top\":[]}"
  Transfer Fcn1 : TransferFcn  Denominator=[1 1]
  Transfer Fcn3 : TransferFcn  Denominator=[1 1]
  Valve2 : SimscapeFluids_lib/Gas/Valves & Orifices/Orifice (G)  orifice_type=foundation.enum.constant_variable.variable  orifice_parameterization=fluids.gas.valves_orifices.enum.OrificeParameterization.Cv  opening_characteristic=fluids.gas.valves_orifices.enum.OpeningCharacteristics.Linear  Cv_constant=4  Cv_max=4  L_Cv_TLU=0 : 0.2 : 1  Cv_TLU=[1e-06, .8, 1.6, 2.4, 3.2, 4]  xT_Cv=0.7  Kv_constant=3.6  Kv_max=3.6  L_Kv_TLU=0 : 0.2 : 1  Kv_TLU=[1e-06, .72, 1.44, 2.16, 2.88, 3.6]  xT_Kv=0.7  C_constant=12 l/(bar*s)  B_crit_constant=0.3  C_max=12 l/(bar*s)  B_crit_linear=0.3  L_C_TLU=0 : 0.2 : 1  C_TLU=[1e-05, 2.4, 4.8, 7.2, 9.6, 12] l/(bar*s)  B_crit_TLU=0.3 * ones(1, 6)  m=0.5  T_ref_C=293.15 K  rho_ref_C=1.185 kg/m^3  orifice_area_constant=1e-4 m^2  orifice_area_max=1e-4 m^2  L_orifice_area_TLU=0 : 0.2 : 1  orifice_area_TLU=[1e-10, 2e-05, 4e-05, 6e-05, 8e-05, .0001] m^2  Cd=0.64  leakage_fraction=1e-6  smoothing_factor=0  B_lam=0.999  area=pi*MV_D ^2/4 m^2
      settings: InternalSimscapePortConfiguration="{\"Bottom\":[],\"Left\":[{\"id\":\"A\",\"label\":\"A\",\"type\":\"foundation.gas.gas\"},{\"id\":\"L\",\"label\":\"L\",\"type\":\"input\"}],\"Right\":[{\"id\":\"B\",\"label\":\"B\",\"type\":\"foundation.gas.gas\"}],\"Top\":[]}"
  Manifold : PMIOPort  Side=Left
  Tank : PMIOPort  Port=2  Side=Right
  wires:
  Transfer Fcn1/1 -> Simulink-PS Converter1/1, Mux2/2
  [Tank_In_cmd] -> Mux1/1, Transfer Fcn3/1
  PS-Simulink Converter4/1 -> Integrator1/1, Scope6/2  "Out"
  Mux2/1 -> Scope5/1
  [Tank_Out_cmd] -> Transfer Fcn1/1, Mux2/1
  Transfer Fcn3/1 -> Simulink-PS Converter3/1, Mux1/2
  Mux1/1 -> Scope5/2
  PS-Simulink Converter2/1 -> Integrator/1, Scope6/1  "In"
  Integrator/1 -> Display/1
  Integrator1/1 -> Display1/1
  connections:
  Manifold/RConn1 -- Manual Valve/LConn1
  PS-Simulink Converter2/LConn1 -- Mass & Energy Flow Rate Sensor (G)1/RConn2
  Simulink-PS Converter3/RConn1 -- Valve2/LConn2
  Check Valve (G)/RConn1 -- Solenoid Valve/LConn1
  Manual Valve/RConn1 -- Mass & Energy Flow Rate Sensor (G)1/LConn1 -- Mass & Energy Flow Rate Sensor (G)3/RConn1
  Check Valve (G)1/RConn1 -- Check Valve (G)/LConn1 -- Tank/RConn1
  PS-Simulink Converter4/LConn1 -- Mass & Energy Flow Rate Sensor (G)3/RConn2
  Mass & Energy Flow Rate Sensor (G)3/LConn1 -- Solenoid Valve/RConn1
  Simulink-PS Converter1/RConn1 -- Solenoid Valve/LConn2
  Valve2/RConn1 -- Check Valve (G)1/LConn1
  Mass & Energy Flow Rate Sensor (G)1/RConn1 -- Valve2/LConn1

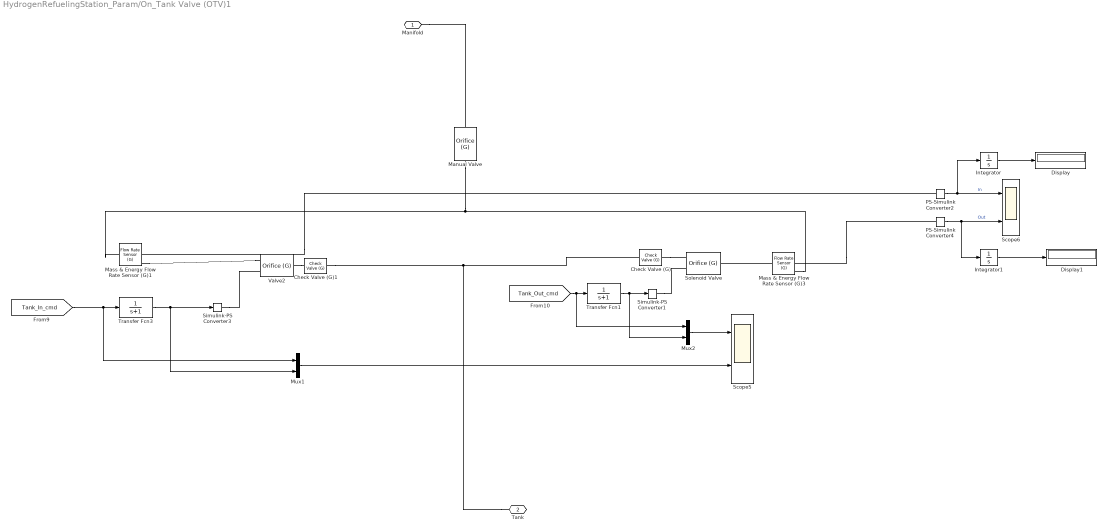
== system HydrogenRefuelingStation_Param/On_Tank Valve (OTV)1 ==
  Check Valve (G) : SimscapeFluids_lib/Gas/Valves & Orifices/Directional Control Valves/Check Valve (G)  opening_pressure_spec=fluids.gas.valves_orifices.enum.PressureControlSpec.PressureA  p_crack_differential=0.01 MPa  p_crack_gauge=1 bar  press_max_differential=70 MPa  press_max_gauge=WP_high bar  valve_parameterization=fluids.gas.valves_orifices.enum.OrificeParameterization.Cv  Cv_max=0.8  xT_Cv=0.7  Kv_max=3.6  xT_Kv=0.7  C_max=12 l/(bar*s)  B_crit_linear=0.3  m=0.5  T_ref_C=293.15 K  rho_ref_C=1.185 kg/m^3  orifice_area_max=1e-4 m^2  Cd=0.64  leakage_fraction=1e-6  smoothing_factor=0.01  B_lam=0.999  area=pi*MV_D ^2/4 m^2
      settings: InternalSimscapePortConfiguration="{\"Bottom\":[],\"Left\":[{\"id\":\"A\",\"label\":\"A\",\"type\":\"foundation.gas.gas\"}],\"Right\":[{\"id\":\"B\",\"label\":\"B\",\"type\":\"foundation.gas.gas\"}],\"Top\":[]}"
  Check Valve (G)1 : SimscapeFluids_lib/Gas/Valves & Orifices/Directional Control Valves/Check Valve (G)  opening_pressure_spec=fluids.gas.valves_orifices.enum.PressureControlSpec.PressureA  p_crack_differential=0.01 MPa  p_crack_gauge=1 bar  press_max_differential=70 MPa  press_max_gauge=WP_high bar  valve_parameterization=fluids.gas.valves_orifices.enum.OrificeParameterization.Cv  Cv_max=0.8  xT_Cv=0.7  Kv_max=3.6  xT_Kv=0.7  C_max=12 l/(bar*s)  B_crit_linear=0.3  m=0.5  T_ref_C=293.15 K  rho_ref_C=1.185 kg/m^3  orifice_area_max=1e-4 m^2  Cd=0.64  leakage_fraction=1e-6  smoothing_factor=0.01  B_lam=0.999  area=pi*MV_D ^2/4 m^2
      settings: InternalSimscapePortConfiguration="{\"Bottom\":[],\"Left\":[{\"id\":\"A\",\"label\":\"A\",\"type\":\"foundation.gas.gas\"}],\"Right\":[{\"id\":\"B\",\"label\":\"B\",\"type\":\"foundation.gas.gas\"}],\"Top\":[]}"
  Display : Display
  Display1 : Display
  Integrator : Integrator
  Integrator1 : Integrator
  Manual Valve : SimscapeFluids_lib/Gas/Valves & Orifices/Orifice (G)  orifice_type=foundation.enum.constant_variable.constant  orifice_parameterization=fluids.gas.valves_orifices.enum.OrificeParameterization.Cv  opening_characteristic=fluids.gas.valves_orifices.enum.OpeningCharacteristics.Linear  Cv_constant=4  Cv_max=4  L_Cv_TLU=0 : 0.2 : 1  Cv_TLU=[1e-06, .8, 1.6, 2.4, 3.2, 4]  xT_Cv=0.7  Kv_constant=3.6  Kv_max=3.6  L_Kv_TLU=0 : 0.2 : 1  Kv_TLU=[1e-06, .72, 1.44, 2.16, 2.88, 3.6]  xT_Kv=0.7  C_constant=12 l/(bar*s)  B_crit_constant=0.3  C_max=12 l/(bar*s)  B_crit_linear=0.3  L_C_TLU=0 : 0.2 : 1  C_TLU=[1e-05, 2.4, 4.8, 7.2, 9.6, 12] l/(bar*s)  B_crit_TLU=0.3 * ones(1, 6)  m=0.5  T_ref_C=293.15 K  rho_ref_C=1.185 kg/m^3  orifice_area_constant=1e-4 m^2  orifice_area_max=1e-4 m^2  L_orifice_area_TLU=0 : 0.2 : 1  orifice_area_TLU=[1e-10, 2e-05, 4e-05, 6e-05, 8e-05, .0001] m^2  Cd=0.64  leakage_fraction=1e-6  smoothing_factor=0  B_lam=0.999  area=pi*inOut_vehTank_D^2/4 m^2
      settings: InternalSimscapePortConfiguration="{\"Bottom\":[],\"Left\":[{\"id\":\"A\",\"label\":\"A\",\"type\":\"foundation.gas.gas\"}],\"Right\":[{\"id\":\"B\",\"label\":\"B\",\"type\":\"foundation.gas.gas\"}],\"Top\":[]}"
  Mass & Energy Flow Rate Sensor (G)1 : fl_lib/Gas/Sensors/Flow Rate Sensor (G)  mass_flow_measure=true  volumetric_flow_measure=false  volumetric_flow_conditions=foundation.enum.volumetric_flow_conditions.actual  p_std=0.101325 MPa  T_std=20 degC  energy_flow_measure=true
      settings: InternalSimscapePortConfiguration="{\"Bottom\":[{\"id\":\"PHI\",\"label\":\"φ\",\"type\":\"output\"}],\"Left\":[{\"id\":\"A\",\"label\":\"A\",\"type\":\"foundation.gas.gas\"}],\"Right\":[{\"id\":\"B\",\"label\":\"B\",\"type\":\"foundation.gas.gas\"},{\"id\":\"M\",\"label\":\"M\",\"type\":\"output\"}],\"Top\":[]}"
  Mass & Energy Flow Rate Sensor (G)3 : fl_lib/Gas/Sensors/Flow Rate Sensor (G)  mass_flow_measure=true  volumetric_flow_measure=false  volumetric_flow_conditions=foundation.enum.volumetric_flow_conditions.actual  p_std=0.101325 MPa  T_std=20 degC  energy_flow_measure=true
      settings: InternalSimscapePortConfiguration="{\"Bottom\":[{\"id\":\"PHI\",\"label\":\"φ\",\"type\":\"output\"}],\"Left\":[{\"id\":\"A\",\"label\":\"A\",\"type\":\"foundation.gas.gas\"}],\"Right\":[{\"id\":\"B\",\"label\":\"B\",\"type\":\"foundation.gas.gas\"},{\"id\":\"M\",\"label\":\"M\",\"type\":\"output\"}],\"Top\":[]}"
  Mux1 : Mux  Inputs=2
  Mux2 : Mux  Inputs=2
  PS-Simulink Converter2 : nesl_utility/PS-Simulink Converter  PhysicalDomain=network_engine_domain  SubClassName=ps_output  LeftPortType=input  RightPortType=output  PseudoPeriodic=off  Frequencies=[]  VectorFormat=inherit  Unit=kg/s  AffineConversion=off
  PS-Simulink Converter4 : nesl_utility/PS-Simulink Converter  PhysicalDomain=network_engine_domain  SubClassName=ps_output  LeftPortType=input  RightPortType=output  PseudoPeriodic=off  Frequencies=[]  VectorFormat=inherit  Unit=kg/s  AffineConversion=off
  Scope5 : Scope  NumInputPorts=2
  Scope6 : Scope  NumInputPorts=2
  Simulink-PS Converter1 : nesl_utility/Simulink-PS Converter  PhysicalDomain=network_engine_domain  SubClassName=ps_input  LeftPortType=input  RightPortType=output  PseudoPeriodic=off  Frequencies=[]  NoiseDistribution=none  NoiseParameters=[]  Unit=1  AffineConversion=off  FilteringAndDerivatives=provide  SimscapeFilterOrder=1  InputFilterTimeConstant=0.001  UdotUserProvided=0
  Simulink-PS Converter3 : nesl_utility/Simulink-PS Converter  PhysicalDomain=network_engine_domain  SubClassName=ps_input  LeftPortType=input  RightPortType=output  PseudoPeriodic=off  Frequencies=[]  NoiseDistribution=none  NoiseParameters=[]  Unit=1  AffineConversion=off  FilteringAndDerivatives=provide  SimscapeFilterOrder=1  InputFilterTimeConstant=0.001  UdotUserProvided=0
  Solenoid Valve : SimscapeFluids_lib/Gas/Valves & Orifices/Orifice (G)  orifice_type=foundation.enum.constant_variable.variable  orifice_parameterization=fluids.gas.valves_orifices.enum.OrificeParameterization.Cv  opening_characteristic=fluids.gas.valves_orifices.enum.OpeningCharacteristics.Linear  Cv_constant=4  Cv_max=4  L_Cv_TLU=0 : 0.2 : 1  Cv_TLU=[1e-06, .8, 1.6, 2.4, 3.2, 4]  xT_Cv=0.7  Kv_constant=3.6  Kv_max=3.6  L_Kv_TLU=0 : 0.2 : 1  Kv_TLU=[1e-06, .72, 1.44, 2.16, 2.88, 3.6]  xT_Kv=0.7  C_constant=12 l/(bar*s)  B_crit_constant=0.3  C_max=12 l/(bar*s)  B_crit_linear=0.3  L_C_TLU=0 : 0.2 : 1  C_TLU=[1e-05, 2.4, 4.8, 7.2, 9.6, 12] l/(bar*s)  B_crit_TLU=0.3 * ones(1, 6)  m=0.5  T_ref_C=293.15 K  rho_ref_C=1.185 kg/m^3  orifice_area_constant=1e-4 m^2  orifice_area_max=1e-4 m^2  L_orifice_area_TLU=0 : 0.2 : 1  orifice_area_TLU=[1e-10, 2e-05, 4e-05, 6e-05, 8e-05, .0001] m^2  Cd=0.64  leakage_fraction=1e-6  smoothing_factor=0  B_lam=0.999  area=pi*SV_D ^2/4 m^2
      settings: InternalSimscapePortConfiguration="{\"Bottom\":[],\"Left\":[{\"id\":\"A\",\"label\":\"A\",\"type\":\"foundation.gas.gas\"},{\"id\":\"L\",\"label\":\"L\",\"type\":\"input\"}],\"Right\":[{\"id\":\"B\",\"label\":\"B\",\"type\":\"foundation.gas.gas\"}],\"Top\":[]}"
  Transfer Fcn1 : TransferFcn  Denominator=[1 1]
  Transfer Fcn3 : TransferFcn  Denominator=[1 1]
  Valve2 : SimscapeFluids_lib/Gas/Valves & Orifices/Orifice (G)  orifice_type=foundation.enum.constant_variable.variable  orifice_parameterization=fluids.gas.valves_orifices.enum.OrificeParameterization.Cv  opening_characteristic=fluids.gas.valves_orifices.enum.OpeningCharacteristics.Linear  Cv_constant=4  Cv_max=4  L_Cv_TLU=0 : 0.2 : 1  Cv_TLU=[1e-06, .8, 1.6, 2.4, 3.2, 4]  xT_Cv=0.7  Kv_constant=3.6  Kv_max=3.6  L_Kv_TLU=0 : 0.2 : 1  Kv_TLU=[1e-06, .72, 1.44, 2.16, 2.88, 3.6]  xT_Kv=0.7  C_constant=12 l/(bar*s)  B_crit_constant=0.3  C_max=12 l/(bar*s)  B_crit_linear=0.3  L_C_TLU=0 : 0.2 : 1  C_TLU=[1e-05, 2.4, 4.8, 7.2, 9.6, 12] l/(bar*s)  B_crit_TLU=0.3 * ones(1, 6)  m=0.5  T_ref_C=293.15 K  rho_ref_C=1.185 kg/m^3  orifice_area_constant=1e-4 m^2  orifice_area_max=1e-4 m^2  L_orifice_area_TLU=0 : 0.2 : 1  orifice_area_TLU=[1e-10, 2e-05, 4e-05, 6e-05, 8e-05, .0001] m^2  Cd=0.64  leakage_fraction=1e-6  smoothing_factor=0  B_lam=0.999  area=pi*MV_D ^2/4 m^2
      settings: InternalSimscapePortConfiguration="{\"Bottom\":[],\"Left\":[{\"id\":\"A\",\"label\":\"A\",\"type\":\"foundation.gas.gas\"},{\"id\":\"L\",\"label\":\"L\",\"type\":\"input\"}],\"Right\":[{\"id\":\"B\",\"label\":\"B\",\"type\":\"foundation.gas.gas\"}],\"Top\":[]}"
  Manifold : PMIOPort  Side=Left
  Tank : PMIOPort  Port=2  Side=Right
  wires:
  Integrator1/1 -> Display1/1
  Integrator/1 -> Display/1
  PS-Simulink Converter2/1 -> Scope6/1, Integrator/1  "In"
  Mux1/1 -> Scope5/2
  Transfer Fcn3/1 -> Mux1/2, Simulink-PS Converter3/1
  [Tank_Out_cmd] -> Mux2/1, Transfer Fcn1/1
  Mux2/1 -> Scope5/1
  PS-Simulink Converter4/1 -> Scope6/2, Integrator1/1  "Out"
  [Tank_In_cmd] -> Transfer Fcn3/1, Mux1/1
  Transfer Fcn1/1 -> Mux2/2, Simulink-PS Converter1/1
  connections:
  Mass & Energy Flow Rate Sensor (G)1/RConn1 -- Valve2/LConn1
  Valve2/RConn1 -- Check Valve (G)1/LConn1
  Simulink-PS Converter1/RConn1 -- Solenoid Valve/LConn2
  Mass & Energy Flow Rate Sensor (G)3/LConn1 -- Solenoid Valve/RConn1
  PS-Simulink Converter4/LConn1 -- Mass & Energy Flow Rate Sensor (G)3/RConn2
  Tank/RConn1 -- Check Valve (G)/LConn1 -- Check Valve (G)1/RConn1
  Mass & Energy Flow Rate Sensor (G)3/RConn1 -- Mass & Energy Flow Rate Sensor (G)1/LConn1 -- Manual Valve/RConn1
  Check Valve (G)/RConn1 -- Solenoid Valve/LConn1
  Simulink-PS Converter3/RConn1 -- Valve2/LConn2
  PS-Simulink Converter2/LConn1 -- Mass & Energy Flow Rate Sensor (G)1/RConn2
  Manifold/RConn1 -- Manual Valve/LConn1
